simulink model "pController"  (R2024a)
settings: Solver=VariableStepAuto  StartTime=0.0  StopTime=20  RelTol=1e-3
model workspace (MAT data in the model file):
  J = 0.00038
  K = 0.028
  KR = 0.1
  L = 0.0001
  R = 5
settings Model: Creator=janho  LastModifiedBy=janho

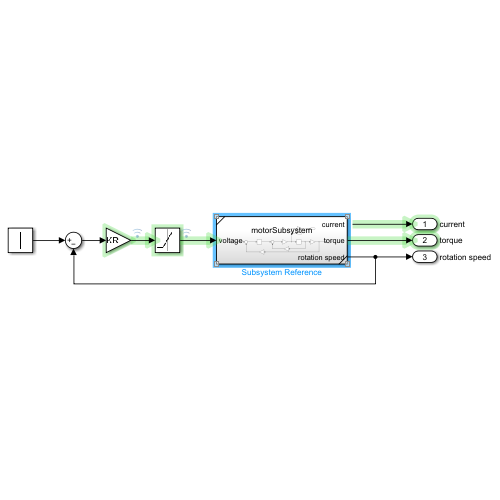
[thumbnail: Simulink's stored preview of the top-level diagram]
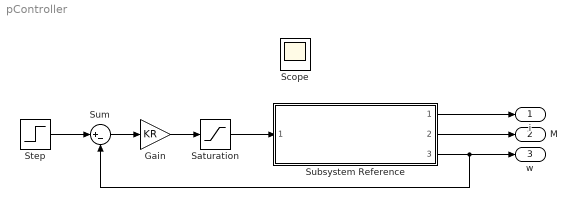
== system pController ==
  Gain : Gain  Gain=KR
  Saturation : Saturate  UpperLimit=10  LowerLimit=-10
  Step : Step  Time=0  After=100  SampleTime=0
  Subsystem Reference : Subsystem  ReferencedSubsystem=motorSubsystem
  Sum : Sum  Inputs=|+-
  i : Outport  SignalName=current
  M : Outport  Port=2  SignalName=torque
  w : Outport  Port=3  SignalName=rotation speed
  Scope : Scope
  wires:
  Step/1 -> Sum/1
  Sum/1 -> Gain/1
  Subsystem Reference/2 -> M/1
  Subsystem Reference/1 -> i/1
  Saturation/1 -> Subsystem Reference/1
  Gain/1 -> Saturation/1
  Subsystem Reference/3 -> w/1, Sum/2
